simulink model "Robust_adaptive_control_WT_Actuator_Fault"  (R2019b)
settings: Solver=VariableStepAuto  StartTime=0.0  StopTime=150  RelTol=1e-3
values from neighbouring files (symbols this model uses):
  af = 5    [PitchActuator_Faults_run.m]
  Alpha = exp(-2*pi*Ts*fc)    [PitchActuator_Faults_run.m]    (also in Test18.mat = 0.990230557066)
  C = [1 0 0 0 0 0;0 0 1 0 0 0;0 0 0 0 1 0]    [PitchActuator_Faults_run.m]
  dwn = 111.7357    [PitchActuator_Faults_run.m]
  dzeta = 10.254    [PitchActuator_Faults_run.m]
  eta = 1    [PitchActuator_Faults_run.m]
  GenEff = 94.4    [Test18.mat]
  k0 = 40    [PitchActuator_Faults_run.m]
  k1 = 61    [PitchActuator_Faults_run.m]
  l0 = [1;1;1]    [PitchActuator_Faults_run.m]
  mu0 = 30    [PitchActuator_Faults_run.m]
  n = 3    [PitchActuator_Faults_run.m]    (also in Test18.mat = 1500)
  omega_0 = w0    (= 1.26710903695)    [PitchActuator_Faults_run.m]
  OutList =     [Test18.mat]
  PC_MaxPit = 1.570796*180/pi    (= 89.999981276)    [PitchActuator_Faults_run.m]    (also in Test18.mat = 1.570796)
  PC_MaxRat = 0.1396263*180/pi    (= 7.99999769903)    [PitchActuator_Faults_run.m]    (also in Test18.mat = 0.1396263)
  PC_MinPit = 0.0    (= 0)    [PitchActuator_Faults_run.m]    (also in Test18.mat)
  R2D = 57.29578    [Test18.mat]
  TqInitial = 43093.5419202    [Test18.mat]
  twozetawn0 = 13.332    [PitchActuator_Faults_run.m]
  VS_CtInSp = 70.16224    [Test18.mat]
  VS_MaxRat = 15000    [Test18.mat]
  VS_MaxTq = 47402.91    [Test18.mat]
  VS_Rgn2K = 2.332287    [Test18.mat]
  VS_RtPwr = 5296610    [Test18.mat]
  VS_Slope15 = 921.830152532    [Test18.mat]
  VS_Slope25 = 3935.03600156    [Test18.mat]
  VS_SySp = 110.618636364    [Test18.mat]
  wgInitial = 122.9096    [Test18.mat]
  wn = 11.11    [PitchActuator_Faults_run.m]
  wn0sqr = 123.4321    [PitchActuator_Faults_run.m]
  wn2 = 5.73    [PitchActuator_Faults_run.m]
undefined symbols (not defined in the file or in its folder): Apb, Apb1, Bpb, Bpb1, sigbuilder_block, strmatch
libraries: simulink_extras x2
settings Model: Creator=samel  LastModifiedBy=samel
settings DebuggingCC: UnderSpecifiedDimensionMsg=warning

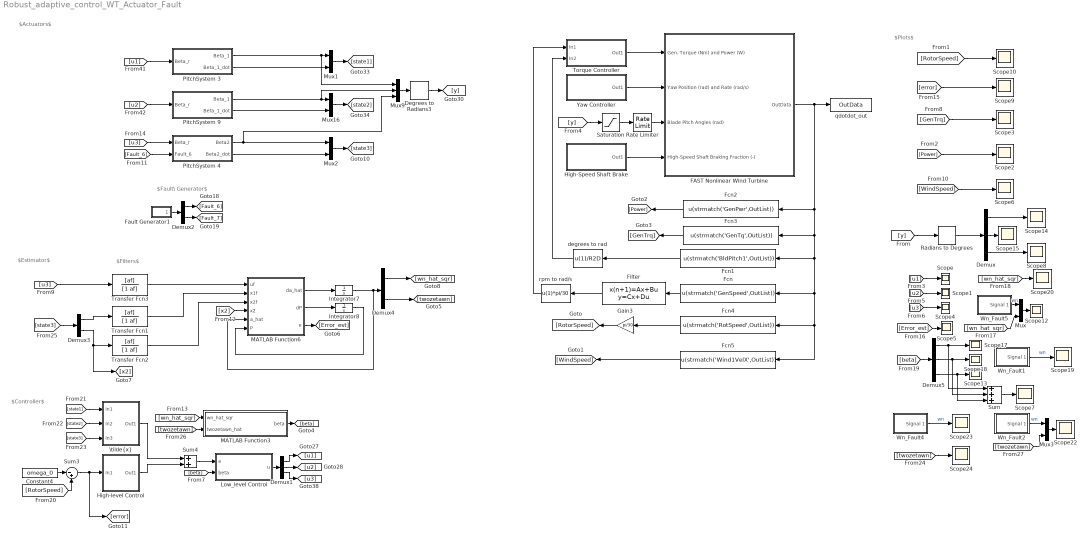
== system Robust_adaptive_control_WT_Actuator_Fault ==
  note: $Estimator$
  note: $Controller$
  note: $Plots$
  note: $Actuators$
  note: $Fault\ Generator$
  note: $Filters$
  Constant4 : Constant  Value=omega_0
  Degrees to Radians3 : simulink_extras/Transformations/Degrees to Radians
  Demux : Demux  Outputs=3
  Demux1 : Demux  Outputs=3
  Demux2 : Demux  Outputs=2
  Demux3 : Demux  Outputs=2
  Demux4 : Demux  Outputs=2
  Demux5 : Demux  Outputs=3
  FAST Nonlinear Wind Turbine : Subsystem  mask(FAST Nonlinear Wind Turbine){}
      mask help: This block contains the FAST S-Function.
      mask init:
      | clear FAST_SFunc
  Fault Generator1 : Subsystem
  Fcn : Fcn  Expr=u(strmatch('GenSpeed',OutList))
  Fcn1 : Fcn  Expr=u(strmatch('BldPitch1',OutList))
  Fcn2 : Fcn  Expr=u(strmatch('GenPwr',OutList))
  Fcn3 : Fcn  Expr=u(strmatch('GenTq',OutList))
  Fcn4 : Fcn  Expr=u(strmatch('RotSpeed',OutList))
  Fcn5 : Fcn  Expr=u(strmatch('Wind1VelX',OutList))
  Filter : DiscreteStateSpace  A=Alpha  B=1 - Alpha  C=Alpha  D=1 - Alpha  InitialCondition=wgInitial  SampleTime=-1
  Gain3 : Gain  Gain=pi/30
  High-Speed Shaft Brake : Subsystem
  High-level Control : Subsystem  mask{Parameter1=on, Parameter2=on}
      mask prompts: Parameter1 "eta"; Parameter2 "k1"
  Integrator7 : Integrator  InitialCondition=[11.11^2;2*0.6*11.11]
  Integrator8 : Integrator  InitialCondition=eye(2)
  Low_level Control : MATLAB Function  TreatAsAtomicUnit=on
  MATLAB Function3 : MATLAB Function  TreatAsAtomicUnit=on
  MATLAB Function6 : MATLAB Function  TreatAsAtomicUnit=on
  Mux{,1..3,16} (5 alike) : Mux  Inputs=2
  Mux9 : Mux  Inputs=3
  PitchSystem 3 : Subsystem
  PitchSystem 4 : Subsystem
  PitchSystem 9 : Subsystem
  Radians to Degrees : simulink_extras/Transformations/Radians to Degrees
  Rate Limiter : RateLimiter  RisingSlewLimit=PC_MaxRat  FallingSlewLimit=-PC_MaxRat  SampleTimeMode=inherited
  Saturation : Saturate  UpperLimit=PC_MaxPit  LowerLimit=PC_MinPit  LinearizeAsGain=off
  Scope{,1..10,12..15,17..20,22..24} (22 alike) : Scope
  Sum : Sum  Inputs=+++
  Sum3 : Sum  Inputs=|-+
  Sum4 : Sum
  Torque Controller : Subsystem
  Transfer Fcn1 : TransferFcn  Numerator=[af]  Denominator=[1 af]
  Transfer Fcn2 : TransferFcn  Numerator=[af]  Denominator=[1 af]
  Transfer Fcn3 : TransferFcn  Numerator=[af]  Denominator=[1 af]
  Wn_Fault1 : Subsystem  Tag=STV Subsys  LoadFcn=sigbuilder_block('load');  StartFcn=sigbuilder_block('start');  StopFcn=sigbuilder_block('stop');  ClipboardFcn=sigbuilder_block('clipboard');  mask(Sigbuilder block){tuvar=[0:10]}
      mask help: Simulink:masks:SigbuilderBlock_MD
      mask init:
      | if ~strcmp(get_param(bdroot(gcbh),'SimulationStatus'),'stopped') tuvar = sigbuilder_block('maskInit'); end
      settings: CopyFcn=sigbuilder_block('copy');  DeleteFcn=sigbuilder_block('delete');  ModelCloseFcn=sigbuilder_block('modelClose');  PreSaveFcn=sigbuilder_block('preSave');  PauseFcn=sigbuilder_block('pause');  ContinueFcn=sigbuilder_block('continue');  NameChangeFcn=sigbuilder_block('namechange');  OpenFcn=sigbuilder_block('open',[1440 -132 1440 723.6 ]);  CloseFcn=sigbuilder_block('close');
      mask Display: plot(0, 0, 100, 100,[2, 2, 32, 32, 2], [68, 8, 8, 68, 68],[32, 2], [38, 38], [32, 19, 2],[53, 60, 44], [32, 17, 17, 2],[16, 16, 31, 31]);txt = getActiveGroup(gcbh);text(2, 100, txt,'verticalAlignment', 'top');
  Wn_Fault2 : Subsystem  Tag=STV Subsys  LoadFcn=sigbuilder_block('load');  StartFcn=sigbuilder_block('start');  StopFcn=sigbuilder_block('stop');  ClipboardFcn=sigbuilder_block('clipboard');  mask(Sigbuilder block){tuvar=[0:10]}
      mask help: Simulink:masks:SigbuilderBlock_MD
      mask init:
      | if ~strcmp(get_param(bdroot(gcbh),'SimulationStatus'),'stopped') tuvar = sigbuilder_block('maskInit'); end
      settings: CopyFcn=sigbuilder_block('copy');  DeleteFcn=sigbuilder_block('delete');  ModelCloseFcn=sigbuilder_block('modelClose');  PreSaveFcn=sigbuilder_block('preSave');  PauseFcn=sigbuilder_block('pause');  ContinueFcn=sigbuilder_block('continue');  NameChangeFcn=sigbuilder_block('namechange');  OpenFcn=sigbuilder_block('open',[5.4 30 1141.2 522.6 ]);  CloseFcn=sigbuilder_block('close');
      mask Display: plot(0, 0, 100, 100,[2, 2, 32, 32, 2], [68, 8, 8, 68, 68],[32, 2], [38, 38], [32, 19, 2],[53, 60, 44], [32, 17, 17, 2],[16, 16, 31, 31]);txt = getActiveGroup(gcbh);text(2, 100, txt,'verticalAlignment', 'top');
  Wn_Fault4 : Subsystem  Tag=STV Subsys  LoadFcn=sigbuilder_block('load');  StartFcn=sigbuilder_block('start');  StopFcn=sigbuilder_block('stop');  ClipboardFcn=sigbuilder_block('clipboard');  mask(Sigbuilder block){tuvar=[0:10]}
      mask help: Simulink:masks:SigbuilderBlock_MD
      mask init:
      | if ~strcmp(get_param(bdroot(gcbh),'SimulationStatus'),'stopped') tuvar = sigbuilder_block('maskInit'); end
      settings: CopyFcn=sigbuilder_block('copy');  DeleteFcn=sigbuilder_block('delete');  ModelCloseFcn=sigbuilder_block('modelClose');  PreSaveFcn=sigbuilder_block('preSave');  PauseFcn=sigbuilder_block('pause');  ContinueFcn=sigbuilder_block('continue');  NameChangeFcn=sigbuilder_block('namechange');  OpenFcn=sigbuilder_block('open',[5.4 30 1141.2 522.6 ]);  CloseFcn=sigbuilder_block('close');
      mask Display: plot(0, 0, 100, 100,[2, 2, 32, 32, 2], [68, 8, 8, 68, 68],[32, 2], [38, 38], [32, 19, 2],[53, 60, 44], [32, 17, 17, 2],[16, 16, 31, 31]);txt = getActiveGroup(gcbh);text(2, 100, txt,'verticalAlignment', 'top');
  Wn_Fault5 : Subsystem  Tag=STV Subsys  LoadFcn=sigbuilder_block('load');  StartFcn=sigbuilder_block('start');  StopFcn=sigbuilder_block('stop');  ClipboardFcn=sigbuilder_block('clipboard');  mask(Sigbuilder block){tuvar=[0:10]}
      mask help: Simulink:masks:SigbuilderBlock_MD
      mask init:
      | if ~strcmp(get_param(bdroot(gcbh),'SimulationStatus'),'stopped') tuvar = sigbuilder_block('maskInit'); end
      settings: CopyFcn=sigbuilder_block('copy');  DeleteFcn=sigbuilder_block('delete');  ModelCloseFcn=sigbuilder_block('modelClose');  PreSaveFcn=sigbuilder_block('preSave');  PauseFcn=sigbuilder_block('pause');  ContinueFcn=sigbuilder_block('continue');  NameChangeFcn=sigbuilder_block('namechange');  OpenFcn=sigbuilder_block('open',[1440 -132 1440 723.6 ]);  CloseFcn=sigbuilder_block('close');
      mask Display: plot(0, 0, 100, 100,[2, 2, 32, 32, 2], [68, 8, 8, 68, 68],[32, 2], [38, 38], [32, 19, 2],[53, 60, 44], [32, 17, 17, 2],[16, 16, 31, 31]);txt = getActiveGroup(gcbh);text(2, 100, txt,'verticalAlignment', 'top');
  Yaw Controller : Subsystem
  "\\tilde{x}" : Subsystem  mask{Beta0=on}
  degrees to rad : Fcn  Expr=u(1)/R2D
  qdotdot_out : ToWorkspace  VariableName=OutData  SampleTime=-1
  rpm to rad/s : Fcn  Expr=u(1)*pi/30
  wires:
  High-Speed Shaft Brake/1(Out1) -> FAST Nonlinear Wind Turbine/4(High-Speed Shaft Braking Fraction (-))
  [WindSpeed] -> Scope6/1
  PitchSystem 3/2(Beta_1_dot) -> Mux1/2
  Demux/3 -> Scope8/1
  PitchSystem 9/2(Beta_1_dot) -> Mux16/2
  Rate Limiter/1 -> FAST Nonlinear Wind Turbine/3(Blade Pitch Angles (rad))
  PitchSystem 3/1("Beta_1 ") -> Mux9/1, Mux1/1
  PitchSystem 9/1("Beta_1 ") -> Mux9/2, Mux16/1
  Mux9/1 -> Degrees to Radians3/1
  rpm to rad/s/1 -> Torque Controller/1(In1)
  Degrees to Radians3/1 -> [y]
  [y] -> Saturation/1
  [error] -> Scope9/1
  Fcn/1 -> Filter/1
  [RotorSpeed] -> Scope10/1
  Fcn2/1 -> [Power]
  [Power] -> Scope2/1
  Radians to Degrees/1 -> Demux/1
  Filter/1 -> rpm to rad/s/1
  [GenTrq] -> Scope3/1
  Gain3/1 -> [RotorSpeed]
  degrees to rad/1 -> Torque Controller/2(In2)
  Fcn3/1 -> [GenTrq]
  Torque Controller/1(Out1) -> FAST Nonlinear Wind Turbine/1(Gen. Torque (Nm) and Power (W))
  Fcn4/1 -> Gain3/1
  Mux1/1 -> [state1]
  Demux/2 -> Scope15/1
  Yaw Controller/1(Out1) -> FAST Nonlinear Wind Turbine/2(Yaw Position (rad) and Rate (rad/s))
  [y] -> Radians to Degrees/1
  FAST Nonlinear Wind Turbine/1(OutData) -> Fcn3/1, Fcn1/1, Fcn5/1, Fcn4/1, Fcn/1, Fcn2/1, qdotdot_out/1
  Fcn5/1 -> [WindSpeed]
  Demux/1 -> Scope14/1
  Saturation/1 -> Rate Limiter/1
  Mux16/1 -> [state2]
  Fcn1/1 -> degrees to rad/1
  Constant4/1 -> Sum3/1
  Sum4/1 -> Low_level Control/1(e)
  [RotorSpeed] -> Sum3/2
  [u1] -> PitchSystem 3/1(Beta_r)
  Fault Generator1/1(Faults) -> Demux2/1
  Demux2/1 -> [Fault_6]
  Demux2/2 -> [Fault_7]
  [u2] -> PitchSystem 9/1(Beta_r)
  [u1] -> Scope/1
  [u3] -> Scope4/1
  [u2] -> Scope1/1
  [state1] -> "\\tilde{x}"/1(In1)
  [state2] -> "\\tilde{x}"/2(In2)
  [state3] -> "\\tilde{x}"/3(In3)
  "\\tilde{x}"/1(Out1) -> Sum4/1
  Sum3/1 -> [error], High-level Control/1(In1)
  High-level Control/1(Out1) -> Sum4/2
  MATLAB Function3/1(beta) -> [beta]
  [u3] -> Transfer Fcn3/1
  [state3] -> Demux3/1
  Demux3/1 -> Transfer Fcn1/1
  Demux3/2 -> [x2], Transfer Fcn2/1
  MATLAB Function6/2(dP) -> Integrator8/1
  Integrator8/1 -> MATLAB Function6/6(P)
  Integrator7/1 -> MATLAB Function6/5(a_hat), Demux4/1
  MATLAB Function6/1(da_hat) -> Integrator7/1
  MATLAB Function6/3(e) -> [Error_est]
  Transfer Fcn3/1 -> MATLAB Function6/1(uf)
  Transfer Fcn1/1 -> MATLAB Function6/2(x1f)
  Transfer Fcn2/1 -> MATLAB Function6/3(x2f)
  [x2] -> MATLAB Function6/4(x2)
  [Error_est] -> Scope5/1
  Wn_Fault5/1(Signal 1) -> Mux/1  "wn"
  [wn_hat_sqr] -> Mux/2
  Mux/1 -> Scope12/1
  Demux4/2 -> [twozetawn]
  Demux5/2 -> Scope18/1, Sum/2
  Demux5/3 -> Scope13/1, Sum/3
  Demux5/1 -> Scope17/1, Sum/1
  [beta] -> Demux5/1
  Demux4/1 -> [wn_hat_sqr]
  Wn_Fault1/1(Signal 1) -> Scope19/1  "wn"
  [wn_hat_sqr] -> Scope20/1
  [Fault_6] -> PitchSystem 4/2(Fault_6)
  Mux2/1 -> [state3]
  PitchSystem 4/1("Beta2 ") -> Mux9/3, Mux2/1
  PitchSystem 4/2("Beta2_dot ") -> Mux2/2
  [u3] -> PitchSystem 4/1(Beta_r)
  Sum/1 -> Scope7/1
  [twozetawn] -> Mux3/2
  Wn_Fault2/1(Signal 1) -> Mux3/1  "wn"
  Mux3/1 -> Scope22/1
  [twozetawn] -> MATLAB Function3/2(twozetawn_hat)
  [wn_hat_sqr] -> MATLAB Function3/1(wn_hat_sqr)
  Wn_Fault4/1(Signal 1) -> Scope23/1  "wn"
  [twozetawn] -> Scope24/1
  Low_level Control/1(u) -> Demux1/1
  Demux1/2 -> [u2]
  Demux1/1 -> [u1]
  Demux1/3 -> [u3]
  [beta] -> Low_level Control/2(beta)

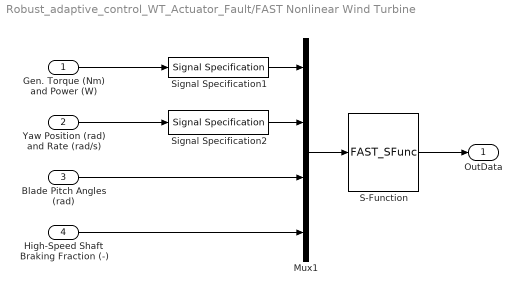
== system Robust_adaptive_control_WT_Actuator_Fault/FAST Nonlinear Wind Turbine ==
  Gen. Torque (Nm) and Power (W) : Inport
  Yaw Position (rad) and Rate (rad/s) : Inport  Port=2
  Blade Pitch Angles (rad) : Inport  Port=3
  High-Speed Shaft Braking Fraction (-) : Inport  Port=4
  Mux1 : Mux
  S-Function : S-Function  FunctionName=FAST_SFunc  Parameters=FAST_InputFileName, TMax, 0  SFunctionDeploymentMode=off  EnableBusSupport=off
  Signal Specification1 : SignalSpecification  OutDataTypeStr=double  Dimensions=2
  Signal Specification2 : SignalSpecification  OutDataTypeStr=double  Dimensions=2
  OutData : Outport  VectorParamsAs1DForOutWhenUnconnected=off
  wires:
  Gen. Torque (Nm) and Power (W)/1 -> Signal Specification1/1
  S-Function/1 -> OutData/1
  Mux1/1 -> S-Function/1
  Blade Pitch Angles (rad)/1 -> Mux1/3
  Yaw Position (rad) and Rate (rad/s)/1 -> Signal Specification2/1
  Signal Specification1/1 -> Mux1/1
  Signal Specification2/1 -> Mux1/2
  High-Speed Shaft Braking Fraction (-)/1 -> Mux1/4

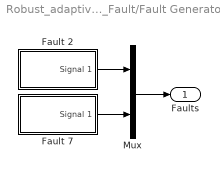
== system Robust_adaptive_control_WT_Actuator_Fault/Fault Generator1 ==
  Fault 2 : Subsystem  Tag=STV Subsys  LoadFcn=sigbuilder_block('load');  StartFcn=sigbuilder_block('start');  StopFcn=sigbuilder_block('stop');  ClipboardFcn=sigbuilder_block('clipboard');  mask(Sigbuilder block){tuvar=[0:10]}
      mask help: Simulink:masks:SigbuilderBlock_MD
      mask init:
      | if ~strcmp(get_param(bdroot(gcbh),'SimulationStatus'),'stopped') tuvar = sigbuilder_block('maskInit'); end
      settings: CopyFcn=sigbuilder_block('copy');  DeleteFcn=sigbuilder_block('delete');  ModelCloseFcn=sigbuilder_block('modelClose');  PreSaveFcn=sigbuilder_block('preSave');  PauseFcn=sigbuilder_block('pause');  ContinueFcn=sigbuilder_block('continue');  NameChangeFcn=sigbuilder_block('namechange');  OpenFcn=sigbuilder_block('open',[5.4 30 1141.2 522.6 ]);  CloseFcn=sigbuilder_block('close');
      mask Display: plot(0, 0, 100, 100,[2, 2, 32, 32, 2], [68, 8, 8, 68, 68],[32, 2], [38, 38], [32, 19, 2],[53, 60, 44], [32, 17, 17, 2],[16, 16, 31, 31]);txt = getActiveGroup(gcbh);text(2, 100, txt,'verticalAlignment', 'top');
  Fault 7 : Subsystem  Tag=STV Subsys  LoadFcn=sigbuilder_block('load');  StartFcn=sigbuilder_block('start');  StopFcn=sigbuilder_block('stop');  ClipboardFcn=sigbuilder_block('clipboard');  mask(Sigbuilder block){tuvar=[0:10]}
      mask help: Simulink:masks:SigbuilderBlock_MD
      mask init:
      | if ~strcmp(get_param(bdroot(gcbh),'SimulationStatus'),'stopped') tuvar = sigbuilder_block('maskInit'); end
      settings: CopyFcn=sigbuilder_block('copy');  DeleteFcn=sigbuilder_block('delete');  ModelCloseFcn=sigbuilder_block('modelClose');  PreSaveFcn=sigbuilder_block('preSave');  PauseFcn=sigbuilder_block('pause');  ContinueFcn=sigbuilder_block('continue');  NameChangeFcn=sigbuilder_block('namechange');  OpenFcn=sigbuilder_block('open',[437.6 199.2 550.4 400 ]);  CloseFcn=sigbuilder_block('close');
      mask Display: plot(0, 0, 100, 100,[2, 2, 32, 32, 2], [68, 8, 8, 68, 68],[32, 2], [38, 38], [32, 19, 2],[53, 60, 44], [32, 17, 17, 2],[16, 16, 31, 31]);txt = getActiveGroup(gcbh);text(2, 100, txt,'verticalAlignment', 'top');
  Mux : Mux  Inputs=2
  Faults : Outport
  wires:
  Fault 7/1(Signal 1) -> Mux/2
  Fault 2/1(Signal 1) -> Mux/1
  Mux/1 -> Faults/1

== system Robust_adaptive_control_WT_Actuator_Fault/High-Speed Shaft Brake ==
  High-Speed Shaft Braking Fraction : Constant  Value=0
  Out1 : Outport  VectorParamsAs1DForOutWhenUnconnected=off
  wires:
  High-Speed Shaft Braking Fraction/1 -> Out1/1

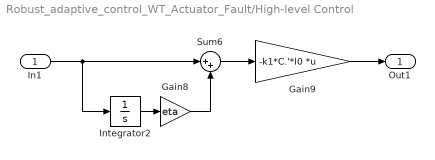
== system Robust_adaptive_control_WT_Actuator_Fault/High-level Control ==
  In1 : Inport
  Gain8 : Gain  Gain=eta
  Gain9 : Gain  Gain=-k1*C.'*l0  Multiplication=Matrix(K*u) (u vector)
  Integrator2 : Integrator
  Sum6 : Sum  Inputs=|++
  Out1 : Outport
  wires:
  Integrator2/1 -> Gain8/1
  Sum6/1 -> Gain9/1
  In1/1 -> Sum6/1, Integrator2/1
  Gain8/1 -> Sum6/2
  Gain9/1 -> Out1/1

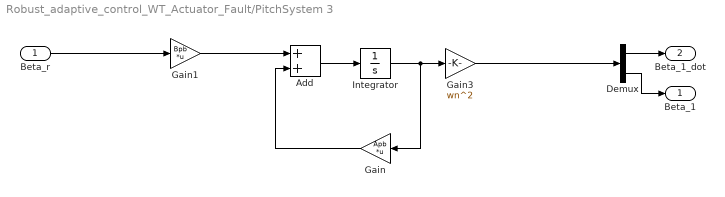
== system Robust_adaptive_control_WT_Actuator_Fault/PitchSystem 3 ==
  Beta_r : Inport
  Add : Sum
  Demux : Demux  Outputs=2
  Gain : Gain  Gain=Apb  Multiplication=Matrix(K*u)
  Gain1 : Gain  Gain=Bpb  Multiplication=Matrix(K*u)
  Gain3 : Gain  Gain=wn^2
  Integrator : Integrator
  "Beta_1 " : Outport
  Beta_1_dot : Outport  Port=2
  wires:
  Gain/1 -> Add/2
  Integrator/1 -> Gain3/1, Gain/1
  Add/1 -> Integrator/1
  Gain1/1 -> Add/1
  Gain3/1 -> Demux/1
  Beta_r/1 -> Gain1/1
  Demux/1 -> Beta_1_dot/1
  Demux/2 -> "Beta_1 "/1

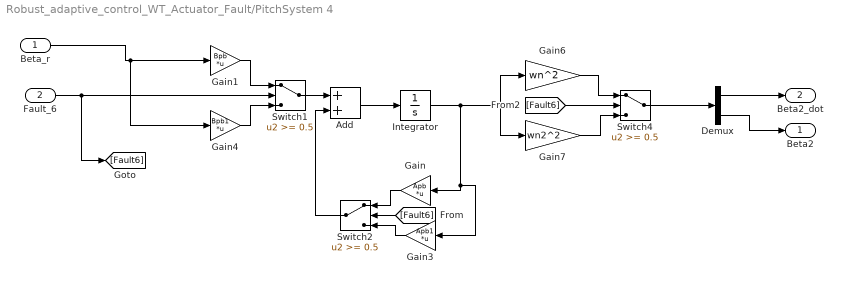
== system Robust_adaptive_control_WT_Actuator_Fault/PitchSystem 4 ==
  Beta_r : Inport
  Fault_6 : Inport  Port=2
  Add : Sum
  Demux : Demux  Outputs=2
  Gain : Gain  Gain=Apb  Multiplication=Matrix(K*u)
  Gain1 : Gain  Gain=Bpb  Multiplication=Matrix(K*u)
  Gain3 : Gain  Gain=Apb1  Multiplication=Matrix(K*u)
  Gain4 : Gain  Gain=Bpb1  Multiplication=Matrix(K*u)
  Gain6 : Gain  Gain=wn^2
  Gain7 : Gain  Gain=wn2^2
  Integrator : Integrator
  Switch1 : Switch  Threshold=0.5
  Switch2 : Switch  Threshold=0.5
  Switch4 : Switch  Threshold=0.5
  "Beta2 " : Outport
  "Beta2_dot " : Outport  Port=2
  wires:
  Integrator/1 -> Gain7/1, Gain6/1, Gain/1, Gain3/1
  Add/1 -> Integrator/1
  Switch1/1 -> Add/1
  Gain1/1 -> Switch1/1
  Gain4/1 -> Switch1/3
  Gain/1 -> Switch2/1
  Gain3/1 -> Switch2/3
  Switch2/1 -> Add/2
  Fault_6/1 -> [Fault6], Switch1/2
  Beta_r/1 -> Gain1/1, Gain4/1
  [Fault6] -> Switch2/2
  [Fault6] -> Switch4/2
  Gain6/1 -> Switch4/1
  Gain7/1 -> Switch4/3
  Switch4/1 -> Demux/1
  Demux/1 -> "Beta2_dot "/1
  Demux/2 -> "Beta2 "/1

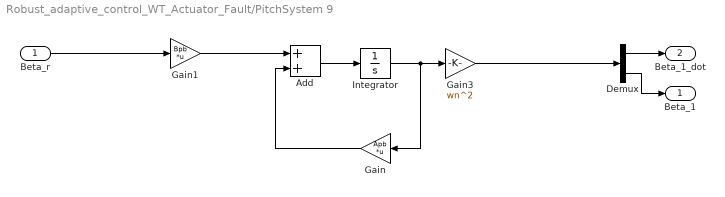
== system Robust_adaptive_control_WT_Actuator_Fault/PitchSystem 9 ==
  Beta_r : Inport
  Add : Sum
  Demux : Demux  Outputs=2
  Gain : Gain  Gain=Apb  Multiplication=Matrix(K*u)
  Gain1 : Gain  Gain=Bpb  Multiplication=Matrix(K*u)
  Gain3 : Gain  Gain=wn^2
  Integrator : Integrator
  "Beta_1 " : Outport
  Beta_1_dot : Outport  Port=2
  wires:
  Gain/1 -> Add/2
  Integrator/1 -> Gain3/1, Gain/1
  Add/1 -> Integrator/1
  Gain1/1 -> Add/1
  Gain3/1 -> Demux/1
  Beta_r/1 -> Gain1/1
  Demux/1 -> Beta_1_dot/1
  Demux/2 -> "Beta_1 "/1

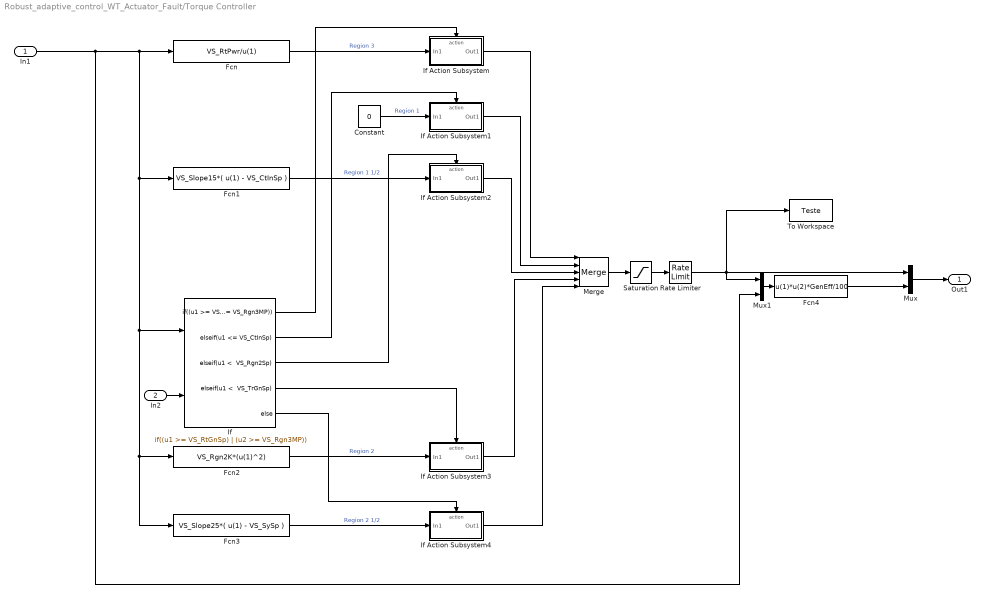
== system Robust_adaptive_control_WT_Actuator_Fault/Torque Controller ==
  In1 : Inport
  In2 : Inport  Port=2
  Constant : Constant  Value=0
  Fcn : Fcn  Expr=VS_RtPwr/u(1)
  Fcn1 : Fcn  Expr=VS_Slope15*( u(1) - VS_CtInSp )
  Fcn2 : Fcn  Expr=VS_Rgn2K*(u(1)^2)
  Fcn3 : Fcn  Expr=VS_Slope25*( u(1) - VS_SySp )
  Fcn4 : Fcn  Expr=u(1)*u(2)*GenEff/100
  If : If  NumInputs=2  IfExpression=(u1 >= VS_RtGnSp) | (u2 >= VS_Rgn3MP)  ElseIfExpressions="u1 <= VS_CtInSp, u1 <  VS_Rgn2Sp, u1 <  VS_TrGnSp"
  If Action Subsystem : Subsystem  TreatAsAtomicUnit=on
  If Action Subsystem1 : Subsystem  TreatAsAtomicUnit=on
  If Action Subsystem2 : Subsystem  TreatAsAtomicUnit=on
  If Action Subsystem3 : Subsystem  TreatAsAtomicUnit=on
  If Action Subsystem4 : Subsystem  TreatAsAtomicUnit=on
  Merge : Merge  Inputs=5  InitialOutput=TqInitial
  Mux : Mux  Inputs=2
  Mux1 : Mux  Inputs=2
  Rate Limiter : RateLimiter  RisingSlewLimit=VS_MaxRat  FallingSlewLimit=-VS_MaxRat  SampleTimeMode=inherited
  Saturation : Saturate  UpperLimit=VS_MaxTq  LowerLimit=0
  To Workspace : ToWorkspace  VariableName=Teste  SaveFormat=Timeseries  SampleTime=-1
  Out1 : Outport  VectorParamsAs1DForOutWhenUnconnected=off
  wires:
  Mux/1 -> Out1/1
  Fcn/1 -> If Action Subsystem/1(In1)  "Region 3"
  If/1 -> If Action Subsystem/Action
  Constant/1 -> If Action Subsystem1/1(In1)  "Region 1"
  If/2 -> If Action Subsystem1/Action
  If/3 -> If Action Subsystem2/Action
  Fcn1/1 -> If Action Subsystem2/1(In1)  "Region 1 1/2"
  If/4 -> If Action Subsystem3/Action
  Fcn2/1 -> If Action Subsystem3/1(In1)  "Region 2"
  If/5 -> If Action Subsystem4/Action
  Fcn3/1 -> If Action Subsystem4/1(In1)  "Region 2 1/2"
  If Action Subsystem/1(Out1) -> Merge/1
  If Action Subsystem1/1(Out1) -> Merge/2
  If Action Subsystem2/1(Out1) -> Merge/3
  If Action Subsystem3/1(Out1) -> Merge/4
  If Action Subsystem4/1(Out1) -> Merge/5
  Mux1/1 -> Fcn4/1
  In1/1 -> Fcn1/1, Fcn2/1, Fcn3/1, If/1, Fcn/1, Mux1/2
  Fcn4/1 -> Mux/2
  Merge/1 -> Saturation/1
  Saturation/1 -> Rate Limiter/1
  In2/1 -> If/2
  Rate Limiter/1 -> To Workspace/1, Mux/1, Mux1/1

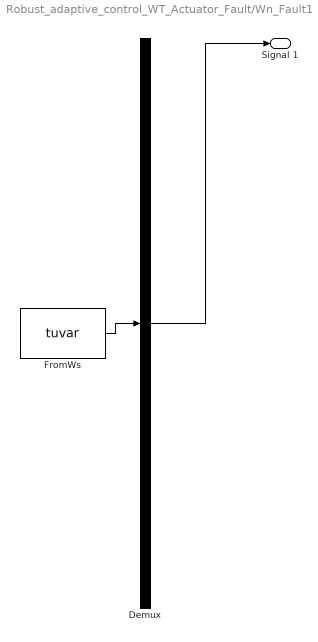
== system Robust_adaptive_control_WT_Actuator_Fault/Wn_Fault1 ==
  Demux : Demux  Tag=STV Demux  Outputs=1
  FromWs : FromWorkspace  Tag=STV FromWs  VariableName=tuvar  SampleTime=0
      SigBuilderData=|
      | common.afterFinalStr = 'Extrapolate'
      | common.sampleTime = 0
      | dataSet.timeRange = [0 600]
      | dataSet.name = 'Group 1'
      | sbobj.Groups.Name = 'Group 1'
      | sbobj.Groups.Signals.Name = 'Signal 1'
      | sbobj.Groups.Signals.XData = [0 50 75 75 124.9 125 600]
      | sbobj.Groups.Signals.YData = [123.4321 123.4321 123.4321 32.8329 32.8329 123.4321 123.4321]
      | sbobj.Groups.TimeRange = [0 600]
  Signal 1 : Outport  Tag=STV Outport  VectorParamsAs1DForOutWhenUnconnected=off
  wires:
  Demux/1 -> Signal 1/1
  FromWs/1 -> Demux/1

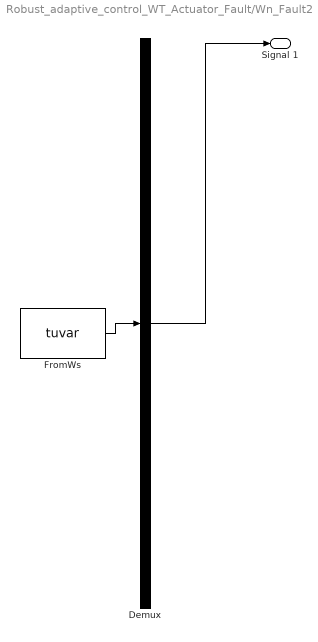
== system Robust_adaptive_control_WT_Actuator_Fault/Wn_Fault2 ==
  Demux : Demux  Tag=STV Demux  Outputs=1
  FromWs : FromWorkspace  Tag=STV FromWs  VariableName=tuvar  SampleTime=0
      SigBuilderData=|
      | common.afterFinalStr = 'Extrapolate'
      | common.sampleTime = 0
      | dataSet.timeRange = [0 600]
      | dataSet.name = 'Group 1'
      | sbobj.Groups.Name = 'Group 1'
      | sbobj.Groups.Signals.Name = 'Signal 1'
      | sbobj.Groups.Signals.XData = [0 50 75 75 124.9 125 600]
      | sbobj.Groups.Signals.YData = [13.332 13.332 13.332 5.157 5.157 13.332 13.332]
      | sbobj.Groups.TimeRange = [0 600]
  Signal 1 : Outport  Tag=STV Outport  VectorParamsAs1DForOutWhenUnconnected=off
  wires:
  Demux/1 -> Signal 1/1
  FromWs/1 -> Demux/1

== system Robust_adaptive_control_WT_Actuator_Fault/Wn_Fault4 ==
  Demux : Demux  Tag=STV Demux  Outputs=1
  FromWs : FromWorkspace  Tag=STV FromWs  VariableName=tuvar  SampleTime=0
      SigBuilderData=|
      | common.afterFinalStr = 'Extrapolate'
      | common.sampleTime = 0
      | dataSet.timeRange = [0 600]
      | dataSet.name = 'Group 1'
      | sbobj.Groups.Name = 'Group 1'
      | sbobj.Groups.Signals.Name = 'Signal 1'
      | sbobj.Groups.Signals.XData = [0 50 75 75 124.9 125 600]
      | sbobj.Groups.Signals.YData = [13.332 13.332 13.332 5.157 5.157 13.332 13.332]
      | sbobj.Groups.TimeRange = [0 600]
  Signal 1 : Outport  Tag=STV Outport  VectorParamsAs1DForOutWhenUnconnected=off
  wires:
  Demux/1 -> Signal 1/1
  FromWs/1 -> Demux/1

== system Robust_adaptive_control_WT_Actuator_Fault/Wn_Fault5 ==
  Demux : Demux  Tag=STV Demux  Outputs=1
  FromWs : FromWorkspace  Tag=STV FromWs  VariableName=tuvar  SampleTime=0
      SigBuilderData=|
      | common.afterFinalStr = 'Extrapolate'
      | common.sampleTime = 0
      | dataSet.timeRange = [0 600]
      | dataSet.name = 'Group 1'
      | sbobj.Groups.Name = 'Group 1'
      | sbobj.Groups.Signals.Name = 'Signal 1'
      | sbobj.Groups.Signals.XData = [0 50 75 75 124.9 125 600]
      | sbobj.Groups.Signals.YData = [123.4321 123.4321 123.4321 32.8329 32.8329 123.4321 123.4321]
      | sbobj.Groups.TimeRange = [0 600]
  Signal 1 : Outport  Tag=STV Outport  VectorParamsAs1DForOutWhenUnconnected=off
  wires:
  Demux/1 -> Signal 1/1
  FromWs/1 -> Demux/1

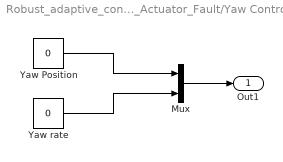
== system Robust_adaptive_control_WT_Actuator_Fault/Yaw Controller ==
  Mux : Mux  Inputs=2
  Yaw Position : Constant  Value=0
  Yaw rate : Constant  Value=0
  Out1 : Outport  VectorParamsAs1DForOutWhenUnconnected=off
  wires:
  Mux/1 -> Out1/1
  Yaw Position/1 -> Mux/1
  Yaw rate/1 -> Mux/2

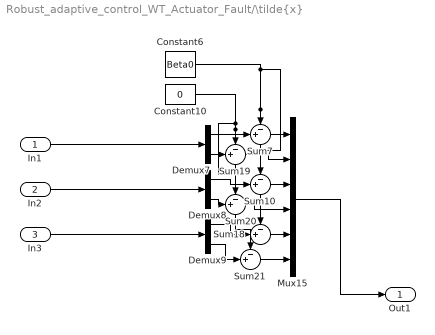
== system Robust_adaptive_control_WT_Actuator_Fault/\tilde{x} ==
  In1 : Inport
  In2 : Inport  Port=2
  In3 : Inport  Port=3
  Constant10 : Constant  Value=0
  Constant6 : Constant  Value=Beta0
  Demux7 : Demux  Outputs=2
  Demux8 : Demux  Outputs=2
  Demux9 : Demux  Outputs=2
  Mux15 : Mux  Inputs=6
  Sum{7,10,18..21} (6 alike) : Sum  Inputs=-+|
  Out1 : Outport
  wires:
  Sum19/1 -> Mux15/2
  In2/1 -> Demux8/1
  Constant10/1 -> Sum21/1, Sum19/1, Sum20/1
  Demux7/2 -> Sum19/2
  Sum7/1 -> Mux15/1
  Constant6/1 -> Sum18/1, Sum7/1, Sum10/1
  Sum18/1 -> Mux15/5
  Sum21/1 -> Mux15/6
  Sum20/1 -> Mux15/4
  Demux7/1 -> Sum7/2
  Demux9/2 -> Sum21/2
  Demux9/1 -> Sum18/2
  Demux8/2 -> Sum20/2
  Demux8/1 -> Sum10/2
  In1/1 -> Demux7/1
  Mux15/1 -> Out1/1
  Sum10/1 -> Mux15/3
  In3/1 -> Demux9/1

== system Robust_adaptive_control_WT_Actuator_Fault/Fault Generator1/Fault 2 ==
  Demux : Demux  Tag=STV Demux  Outputs=1
  FromWs : FromWorkspace  Tag=STV FromWs  VariableName=tuvar  SampleTime=0
      SigBuilderData=|
      | common.afterFinalStr = 'Extrapolate'
      | common.sampleTime = 0
      | dataSet.timeRange = [0 600]
      | dataSet.name = 'Group 1'
      | sbobj.Groups.Name = 'Group 1'
      | sbobj.Groups.Signals.Name = 'Signal 1'
      | sbobj.Groups.Signals.XData = [0 75 75 125 125 600]
      | sbobj.Groups.Signals.YData = [1 1 0 0 1 1]
      | sbobj.Groups.TimeRange = [0 600]
  Signal 1 : Outport  Tag=STV Outport
  wires:
  Demux/1 -> Signal 1/1
  FromWs/1 -> Demux/1

== system Robust_adaptive_control_WT_Actuator_Fault/Fault Generator1/Fault 7 ==
  Demux : Demux  Tag=STV Demux  Outputs=1
  FromWs : FromWorkspace  Tag=STV FromWs  VariableName=tuvar  SampleTime=0
      SigBuilderData=|
      | common.afterFinalStr = 'Extrapolate'
      | common.sampleTime = 0
      | dataSet.timeRange = [0 800]
      | dataSet.name = 'Group 1'
      | sbobj.Groups.Name = 'Group 1'
      | sbobj.Groups.Signals.Name = 'Signal 1'
      | sbobj.Groups.Signals.XData = [0 150 180 220 250 800]
      | sbobj.Groups.Signals.YData = [1 1 0 0 1 1]
      | sbobj.Groups.TimeRange = [0 800]
  Signal 1 : Outport  Tag=STV Outport
  wires:
  Demux/1 -> Signal 1/1
  FromWs/1 -> Demux/1

== system Robust_adaptive_control_WT_Actuator_Fault/Torque Controller/If Action Subsystem ==
  In1 : Inport
  Action Port : ActionPort  ActionPortLabel=if((u1 >= VS_RtGnSp) | (u2 >= VS_Rgn3MP))
  Out1 : Outport  VectorParamsAs1DForOutWhenUnconnected=off
  wires:
  In1/1 -> Out1/1

== system Robust_adaptive_control_WT_Actuator_Fault/Torque Controller/If Action Subsystem1 ==
  In1 : Inport
  Action Port : ActionPort  ActionPortLabel=elseif(u1 <= VS_CtInSp)
  Out1 : Outport  VectorParamsAs1DForOutWhenUnconnected=off
  wires:
  In1/1 -> Out1/1

== system Robust_adaptive_control_WT_Actuator_Fault/Torque Controller/If Action Subsystem2 ==
  In1 : Inport
  Action Port : ActionPort  ActionPortLabel="elseif( u1 <  VS_Rgn2Sp)"
  Out1 : Outport  VectorParamsAs1DForOutWhenUnconnected=off
  wires:
  In1/1 -> Out1/1

== system Robust_adaptive_control_WT_Actuator_Fault/Torque Controller/If Action Subsystem3 ==
  In1 : Inport
  Action Port : ActionPort  ActionPortLabel="elseif( u1 <  VS_TrGnSp)"
  Out1 : Outport  VectorParamsAs1DForOutWhenUnconnected=off
  wires:
  In1/1 -> Out1/1

== system Robust_adaptive_control_WT_Actuator_Fault/Torque Controller/If Action Subsystem4 ==
  In1 : Inport
  Action Port : ActionPort  ActionPortLabel=else
  Out1 : Outport  VectorParamsAs1DForOutWhenUnconnected=off
  wires:
  In1/1 -> Out1/1

== matlab function Robust_adaptive_control_WT_Actuator_Fault/Low_level Control ==
  data: e input; u output; k2 parameter; beta input
function u    = fcn(e,k2,beta)
u            =  -beta*k2.'*e;

== matlab function Robust_adaptive_control_WT_Actuator_Fault/MATLAB Function3 ==
  data: beta output; wn_hat_sqr input; twozetawn0 parameter; dwn parameter; dzeta parameter; wn0sqr parameter; twozetawn_hat input; n parameter
function beta   = fcn(wn_hat_sqr,twozetawn0,dwn,dzeta, wn0sqr, twozetawn_hat,n)

theta      =  0.5*(abs(wn0sqr-wn_hat_sqr)/dwn+abs(twozetawn0-twozetawn_hat)/dzeta); %Fault mapping indicator
beta       =  1/n*[1+0.5*theta;1+0.5*theta;1-theta];                                %Splitter

== matlab function Robust_adaptive_control_WT_Actuator_Fault/MATLAB Function6 ==
  data: uf input; da_hat output; x1f input; x2f input; x2 input; a_hat input; P input; dP output; e output; mu0 parameter; k0 parameter; af parameter
function [da_hat,dP,e] = fcn(uf,x1f,x2f,x2,a_hat,P,mu0,k0,af)

mu  =   mu0*(1-norm(P)/k0);    % Bounded gain forgetting factor technique 
w       =   [uf-x1f -x2f];        % Regressor
dP      =   mu*P-P*(w.')*w*P; % Matrix gain (Estimation convariance matrix)
y       =   af*x2-af*x2f;         % Measurement output
e       =   w*a_hat-y;            % Prediction error
da_hat  =   -P*(w.')*e;           % Update law for parameter estimation
